simulink model "control_tests"  (R2023b)
settings: Solver=VariableStepAuto  StartTime=0.0  StopTime=30  RelTol=1e-3
values from neighbouring files (symbols this model uses):
  Bp_ = 1.25e-5    (= 1.25e-05)    [stable_pendulum_model.m]
  g_ = 9.81    [stable_pendulum_model.m]
  Jp_ = (1/12)*mp_*(3*rp^2 + Lp^2)    (= 3.3718538025e-05)    [stable_pendulum_model.m]
  Jr_ex_ = 9.5e-5    (= 9.5e-05)    [stable_pendulum_model.m]
  Kc_ = 0.042    [stable_pendulum_model.m]
  Ke_ = 0.042    [stable_pendulum_model.m]
  lp_ = 0.95*Lp/2    (= 0.061275)    [stable_pendulum_model.m]
  Lr_ = 0.09    [stable_pendulum_model.m]
  mp_ = 0.02421    [stable_pendulum_model.m]
  Ra_ = 8.4    [stable_pendulum_model.m]
  theta_0 = 0    [stable_pendulum_model.m]
libraries: cstblocks x3
settings Model: Creator=renzo  LastModifiedBy=renzo

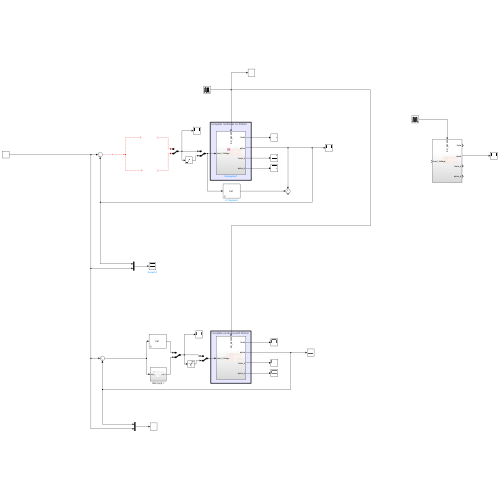
[thumbnail: Simulink's stored preview of the top-level diagram]
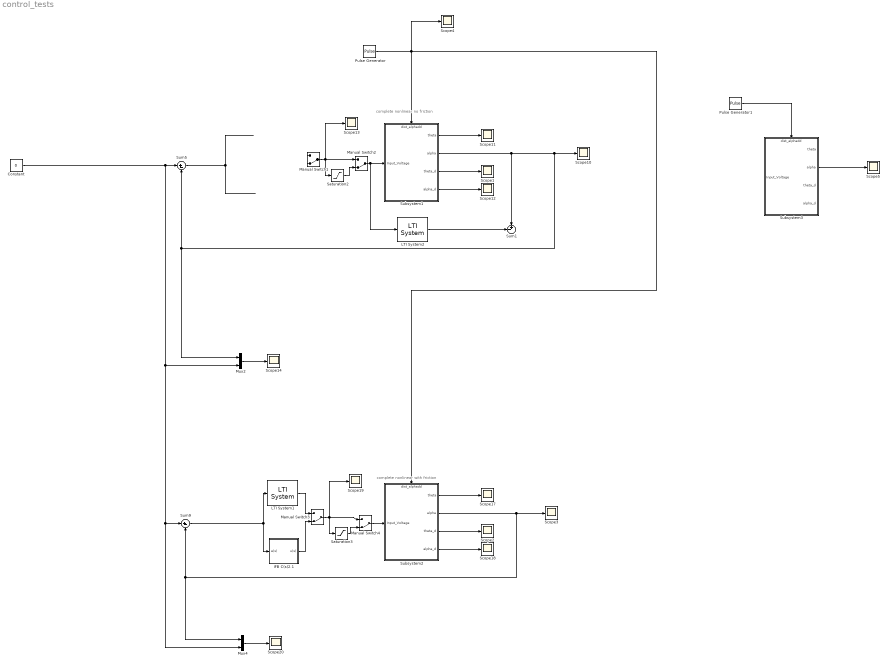
== system control_tests ==
  note: complete nonlinear no friction
  note: complete nonlinear with friction
  Constant : Constant  Value=0
  IFB C(s)2.1 : Subsystem
  LTI System1 : cstblocks/LTI System  sys=Cs1  IC=[]  PadeOrder=0
  LTI System2 : cstblocks/LTI System  sys=Cs1  IC=[]  PadeOrder=0
  Manual Switch{1..4} (4 alike) : ManualSwitch  CurrentSetting=0
  Mux2 : Mux  Inputs=2
  Mux4 : Mux  Inputs=2
  Pulse Generator : DiscretePulseGenerator  PulseType=Time based  Amplitude=20  Period=7  PulseWidth=5  PhaseDelay=3
  Pulse Generator1 : DiscretePulseGenerator  PulseType=Time based  Amplitude=20  Period=7  PulseWidth=5  PhaseDelay=3
  Saturation2 : Saturate  UpperLimit=10  LowerLimit=-10
  Saturation3 : Saturate  UpperLimit=10  LowerLimit=-10
  Scope{1..5,10..14,17..20} (14 alike) : Scope
  Subsystem1 : Subsystem
      settings: PortSchema="{\"entries\":[{\"content\":{\"sides\":[{\"content\":{\"connectorIds\":[\"In1\"]},\"type\":\"ConnectorPlacement.EquallySpacedRectSide\",\"uuid\":\"871ba934-2a41-428b-821f-daa366d85b89\"},{\"content\":{\"connectorIds\":[\"Out1\",\"Out2\",\"Out3\",\"Out4\"],\"side\":\"RIGHT\"},\"type\":\"ConnectorPlacement.EquallySpacedRectSide\",\"uuid\":\"80e9fc77-4911-4b7a-8bf9-66ec4cab57cc\"},{\"content\":{\"connectorIds\":[\"In2\"],\"side\":\"TOP\"},\"type\":\"ConnectorPlacement.EquallySpacedRectSide\",\"uuid\":\"5ed9de82-5230-4695-8afb-09027cc7b06e\"}]},\"type\":\"ConnectorPlacement.EquallySpacedConnector\",\"uuid\":\"352cd2d9-0c64-485c-bb70-89dea2777168\"}],\"packageUris\":[\"http://schema.mathworks.com/mf0/Connector/R2020b\"],\"version\":\"1.0\"}"
  Subsystem2 : Subsystem
      settings: PortSchema="{\"entries\":[{\"content\":{\"sides\":[{\"content\":{\"connectorIds\":[\"In1\"]},\"type\":\"ConnectorPlacement.EquallySpacedRectSide\",\"uuid\":\"871ba934-2a41-428b-821f-daa366d85b89\"},{\"content\":{\"connectorIds\":[\"Out1\",\"Out2\",\"Out3\",\"Out4\"],\"side\":\"RIGHT\"},\"type\":\"ConnectorPlacement.EquallySpacedRectSide\",\"uuid\":\"80e9fc77-4911-4b7a-8bf9-66ec4cab57cc\"},{\"content\":{\"connectorIds\":[\"In2\"],\"side\":\"TOP\"},\"type\":\"ConnectorPlacement.EquallySpacedRectSide\",\"uuid\":\"5ed9de82-5230-4695-8afb-09027cc7b06e\"}]},\"type\":\"ConnectorPlacement.EquallySpacedConnector\",\"uuid\":\"352cd2d9-0c64-485c-bb70-89dea2777168\"}],\"packageUris\":[\"http://schema.mathworks.com/mf0/Connector/R2020b\"],\"version\":\"1.0\"}"
  Subsystem3 : Subsystem
      settings: PortSchema="{\"entries\":[{\"content\":{\"sides\":[{\"content\":{\"connectorIds\":[\"In1\"]},\"type\":\"ConnectorPlacement.EquallySpacedRectSide\",\"uuid\":\"871ba934-2a41-428b-821f-daa366d85b89\"},{\"content\":{\"connectorIds\":[\"Out1\",\"Out2\",\"Out3\",\"Out4\"],\"side\":\"RIGHT\"},\"type\":\"ConnectorPlacement.EquallySpacedRectSide\",\"uuid\":\"80e9fc77-4911-4b7a-8bf9-66ec4cab57cc\"},{\"content\":{\"connectorIds\":[\"In2\"],\"side\":\"TOP\"},\"type\":\"ConnectorPlacement.EquallySpacedRectSide\",\"uuid\":\"5ed9de82-5230-4695-8afb-09027cc7b06e\"}]},\"type\":\"ConnectorPlacement.EquallySpacedConnector\",\"uuid\":\"352cd2d9-0c64-485c-bb70-89dea2777168\"}],\"packageUris\":[\"http://schema.mathworks.com/mf0/Connector/R2020b\"],\"version\":\"1.0\"}"
  Sum1 : Sum  Inputs=-+|
  Sum5 : Sum  Inputs=|+-
  Sum9 : Sum  Inputs=|+-
  wires:
  Mux4/1 -> Scope20/1
  Mux2/1 -> Scope14/1
  Constant/1 -> Mux4/2, Sum9/1, Mux2/2, Sum5/1
  Sum9/1 -> LTI System1/1, IFB C(s)2.1/1(e(s))
  LTI System1/1 -> Manual Switch3/1
  Subsystem1/2(alpha) -> Sum1/2, Sum5/2, Mux2/1, Scope10/1
  Manual Switch4/1 -> Subsystem2/1(Input_Voltage)
  Manual Switch2/1 -> LTI System2/1, Subsystem1/1(Input_Voltage)
  Saturation2/1 -> Manual Switch2/2
  ? -> Manual Switch1/1
  ? -> Manual Switch1/2
  Subsystem2/2(alpha) -> Scope3/1, Sum9/2, Mux4/1
  Subsystem2/1(theta) -> Scope17/1
  IFB C(s)2.1/1(u(s)) -> Manual Switch3/2
  Subsystem2/4(alpha_d) -> Scope18/1
  Manual Switch1/1 -> Saturation2/1, Manual Switch2/1, Scope13/1
  Saturation3/1 -> Manual Switch4/2
  Subsystem1/4(alpha_d) -> Scope12/1
  Manual Switch3/1 -> Saturation3/1, Manual Switch4/1, Scope19/1
  Subsystem1/3(theta_d) -> Scope1/1
  Subsystem1/1(theta) -> Scope11/1
  Sum5/1 -> ?
  Subsystem2/3(theta_d) -> Scope2/1
  Pulse Generator/1 -> Scope4/1, Subsystem2/2(dist_alphadd), Subsystem1/2(dist_alphadd)
  Pulse Generator1/1 -> Subsystem3/2(dist_alphadd)
  Subsystem3/2(alpha) -> Scope5/1
  LTI System2/1 -> Sum1/1

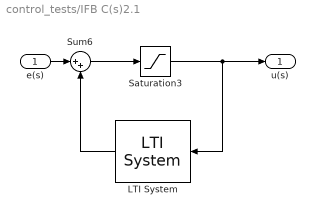
== system control_tests/IFB C(s)2.1 ==
  e(s) : Inport
  LTI System : cstblocks/LTI System  sys=Hs1  IC=[]  PadeOrder=0
  Saturation3 : Saturate  UpperLimit=10  LowerLimit=-10
  Sum6 : Sum  Inputs=|++
  u(s) : Outport
  wires:
  LTI System/1 -> Sum6/2
  Sum6/1 -> Saturation3/1
  Saturation3/1 -> u(s)/1, LTI System/1
  e(s)/1 -> Sum6/1

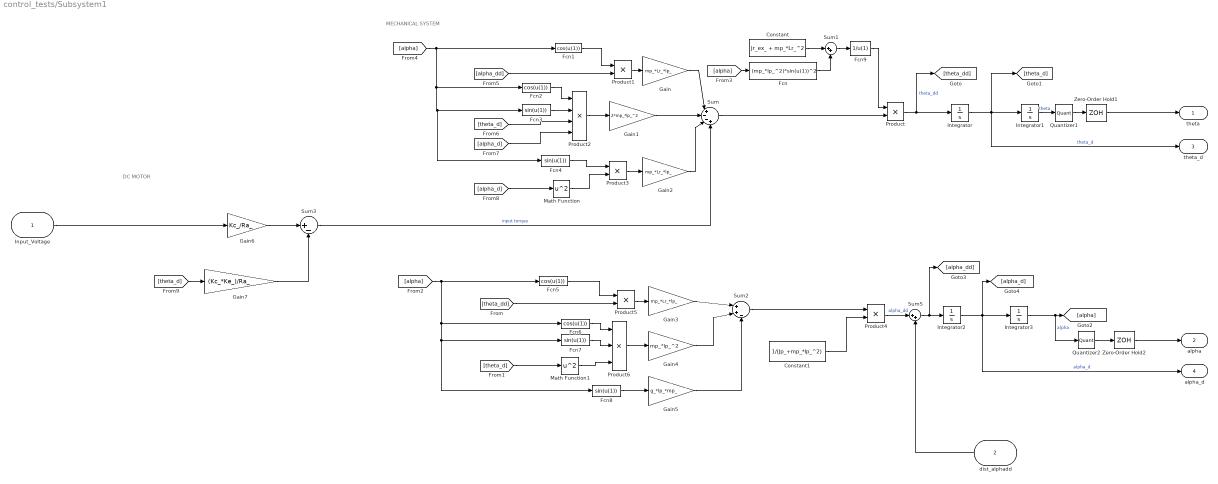
== system control_tests/Subsystem1 ==
  note: DC MOTOR
  note: MECHANICAL SYSTEM
  Input_Voltage : Inport
  dist_alphadd : Inport  Port=2
  Constant : Constant  Value=Jr_ex_ + mp_*Lr_^2
  Constant1 : Constant  Value=1/(Jp_+mp_*lp_^2)
  Fcn : Fcn  Expr=(mp_*lp_^2)*sin(u(1))^2
  Fcn{1..2,5..6} (4 alike) : Fcn  Expr=cos(u(1))
  Fcn{3..4,7..8} (4 alike) : Fcn  Expr=sin(u(1))
  Fcn9 : Fcn  Expr=1/u(1)
  Gain : Gain  Gain=mp_*Lr_*lp_
  Gain1 : Gain  Gain=2*mp_*lp_^2
  Gain2 : Gain  Gain=mp_*Lr_*lp_
  Gain3 : Gain  Gain=mp_*Lr_*lp_
  Gain4 : Gain  Gain=mp_*lp_^2
  Gain5 : Gain  Gain=g_*lp_*mp_
  Gain6 : Gain  Gain=Kc_/Ra_
  Gain7 : Gain  Gain=(Kc_*Ke_)/Ra_
  Integrator : Integrator
  Integrator1 : Integrator  InitialCondition=theta_0
  Integrator2 : Integrator
  Integrator3 : Integrator
  Math Function : Math  Operator=square
  Math Function1 : Math  Operator=square
  Product{,1,3..5} (5 alike) : Product
  Product2 : Product  Inputs=4
  Product6 : Product  Inputs=3
  Quantizer1 : Quantizer  QuantizationInterval=0.0037
  Quantizer2 : Quantizer  QuantizationInterval=0.0037
  Sum : Sum  Inputs=|+--+
  Sum1 : Sum  Inputs=|++
  Sum2 : Sum  Inputs=|++-
  Sum3 : Sum  Inputs=|+-
  Sum5 : Sum  Inputs=|++
  Zero-Order Hold1 : ZeroOrderHold  SampleTime=2e-3
  Zero-Order Hold2 : ZeroOrderHold  SampleTime=2e-3
  theta : Outport
  alpha : Outport  Port=2
  theta_d : Outport  Port=3
  alpha_d : Outport  Port=4
  wires:
  Integrator2/1 -> alpha_d/1, Integrator3/1, [alpha_d]  "alpha_d"
  Fcn6/1 -> Product6/1
  Product4/1 -> Sum5/1  "alpha_dd"
  Fcn4/1 -> Product3/1
  Integrator/1 -> theta_d/1, [theta_d], Integrator1/1  "theta_d"
  Gain1/1 -> Sum/2
  Gain6/1 -> Sum3/1
  Fcn3/1 -> Product2/2
  Fcn1/1 -> Product1/1
  Integrator1/1 -> Quantizer1/1  "theta"
  Fcn8/1 -> Gain5/1
  Fcn7/1 -> Product6/2
  Gain5/1 -> Sum2/3
  Sum1/1 -> Fcn9/1
  Fcn/1 -> Sum1/2
  Product1/1 -> Gain/1
  Fcn9/1 -> Product/1
  Product3/1 -> Gain2/1
  Sum/1 -> Product/2
  [alpha_d] -> Math Function/1
  [theta_dd] -> Product5/2
  [theta_d] -> Gain7/1
  Product5/1 -> Gain3/1
  Fcn5/1 -> Product5/1
  Product6/1 -> Gain4/1
  Sum2/1 -> Product4/1
  Math Function1/1 -> Product6/3
  Math Function/1 -> Product3/2
  Product/1 -> Integrator/1, [theta_dd]  "theta_dd"
  Gain4/1 -> Sum2/2
  Input_Voltage/1 -> Gain6/1
  Constant/1 -> Sum1/1
  [alpha] -> Fcn8/1, Fcn7/1, Fcn6/1, Fcn5/1
  Constant1/1 -> Product4/2
  Product2/1 -> Gain1/1
  [alpha] -> Fcn4/1, Fcn3/1, Fcn2/1, Fcn1/1
  [alpha_d] -> Product2/4
  [alpha_dd] -> Product1/2
  [alpha] -> Fcn/1
  Fcn2/1 -> Product2/1
  Sum3/1 -> Sum/4  "input torque"
  Gain2/1 -> Sum/3
  Gain/1 -> Sum/1
  Gain3/1 -> Sum2/1
  [theta_d] -> Math Function1/1
  Gain7/1 -> Sum3/2
  [theta_d] -> Product2/3
  Quantizer1/1 -> Zero-Order Hold1/1
  Zero-Order Hold1/1 -> theta/1
  Quantizer2/1 -> Zero-Order Hold2/1
  Zero-Order Hold2/1 -> alpha/1
  Integrator3/1 -> Quantizer2/1, [alpha]  "alpha"
  Sum5/1 -> [alpha_dd], Integrator2/1
  dist_alphadd/1 -> Sum5/2

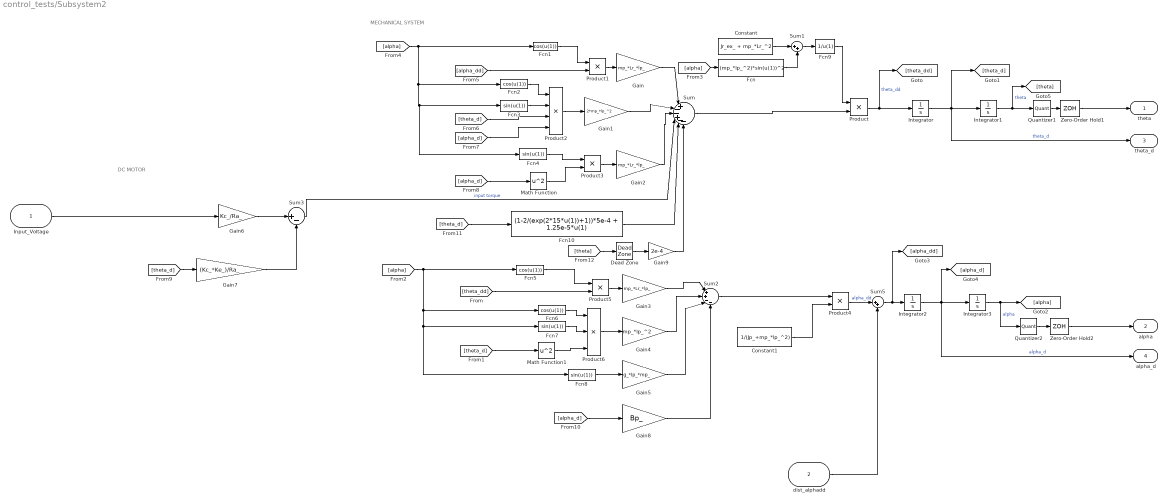
== system control_tests/Subsystem2 ==
  note: MECHANICAL SYSTEM
  note: DC MOTOR
  Input_Voltage : Inport
  dist_alphadd : Inport  Port=2
  Constant : Constant  Value=Jr_ex_ + mp_*Lr_^2
  Constant1 : Constant  Value=1/(Jp_+mp_*lp_^2)
  Dead Zone : DeadZone  LowerValue=0  UpperValue=0  ZeroCross=off
  Fcn : Fcn  Expr=(mp_*lp_^2)*sin(u(1))^2
  Fcn{1..2,5..6} (4 alike) : Fcn  Expr=cos(u(1))
  Fcn10 : Fcn  Expr=(1-2/(exp(2*15*u(1))+1))*5e-4 + 1.25e-5*u(1)
  Fcn{3..4,7..8} (4 alike) : Fcn  Expr=sin(u(1))
  Fcn9 : Fcn  Expr=1/u(1)
  Gain : Gain  Gain=mp_*Lr_*lp_
  Gain1 : Gain  Gain=2*mp_*lp_^2
  Gain2 : Gain  Gain=mp_*Lr_*lp_
  Gain3 : Gain  Gain=mp_*Lr_*lp_
  Gain4 : Gain  Gain=mp_*lp_^2
  Gain5 : Gain  Gain=g_*lp_*mp_
  Gain6 : Gain  Gain=Kc_/Ra_
  Gain7 : Gain  Gain=(Kc_*Ke_)/Ra_
  Gain8 : Gain  Gain=Bp_
  Gain9 : Gain  Gain=2e-4
  Integrator{,1..3} (4 alike) : Integrator
  Math Function : Math  Operator=square
  Math Function1 : Math  Operator=square
  Product{,1,3..5} (5 alike) : Product
  Product2 : Product  Inputs=4
  Product6 : Product  Inputs=3
  Quantizer1 : Quantizer  QuantizationInterval=0.0037
  Quantizer2 : Quantizer  QuantizationInterval=0.0037
  Sum : Sum  Inputs=|+--+--
  Sum1 : Sum  Inputs=|++
  Sum2 : Sum  Inputs=|++--
  Sum3 : Sum  Inputs=|+-
  Sum5 : Sum  Inputs=|++
  Zero-Order Hold1 : ZeroOrderHold  SampleTime=2e-3
  Zero-Order Hold2 : ZeroOrderHold  SampleTime=2e-3
  theta : Outport
  alpha : Outport  Port=2
  theta_d : Outport  Port=3
  alpha_d : Outport  Port=4
  wires:
  [theta_d] -> Product2/3
  Gain7/1 -> Sum3/2
  [theta_d] -> Math Function1/1
  Gain3/1 -> Sum2/1
  Gain/1 -> Sum/1
  Gain2/1 -> Sum/3
  Sum3/1 -> Sum/4  "input torque"
  Fcn2/1 -> Product2/1
  [alpha] -> Fcn/1
  [alpha_dd] -> Product1/2
  [alpha_d] -> Product2/4
  [alpha] -> Fcn1/1, Fcn2/1, Fcn3/1, Fcn4/1
  Product2/1 -> Gain1/1
  Constant1/1 -> Product4/2
  [alpha] -> Fcn5/1, Fcn6/1, Fcn7/1, Fcn8/1
  Constant/1 -> Sum1/1
  Input_Voltage/1 -> Gain6/1
  Gain4/1 -> Sum2/2
  Product/1 -> [theta_dd], Integrator/1  "theta_dd"
  Math Function/1 -> Product3/2
  Math Function1/1 -> Product6/3
  Sum2/1 -> Product4/1
  Product6/1 -> Gain4/1
  Fcn5/1 -> Product5/1
  Integrator3/1 -> [alpha], Quantizer2/1  "alpha"
  Product5/1 -> Gain3/1
  [theta_d] -> Gain7/1
  [theta_dd] -> Product5/2
  [alpha_d] -> Math Function/1
  Sum/1 -> Product/2
  Product3/1 -> Gain2/1
  Fcn9/1 -> Product/1
  Product1/1 -> Gain/1
  Fcn/1 -> Sum1/2
  Sum1/1 -> Fcn9/1
  Gain5/1 -> Sum2/3
  Fcn7/1 -> Product6/2
  Fcn8/1 -> Gain5/1
  Integrator1/1 -> Quantizer1/1, [theta]  "theta"
  Fcn1/1 -> Product1/1
  Fcn3/1 -> Product2/2
  Gain6/1 -> Sum3/1
  Gain1/1 -> Sum/2
  Integrator/1 -> Integrator1/1, [theta_d], theta_d/1  "theta_d"
  Fcn4/1 -> Product3/1
  Product4/1 -> Sum5/1  "alpha_dd"
  Fcn6/1 -> Product6/1
  Integrator2/1 -> [alpha_d], Integrator3/1, alpha_d/1  "alpha_d"
  [alpha_d] -> Gain8/1
  Gain8/1 -> Sum2/4
  [theta_d] -> Fcn10/1
  Dead Zone/1 -> Gain9/1
  Gain9/1 -> Sum/6
  [theta] -> Dead Zone/1
  Fcn10/1 -> Sum/5
  Quantizer1/1 -> Zero-Order Hold1/1
  Zero-Order Hold1/1 -> theta/1
  Quantizer2/1 -> Zero-Order Hold2/1
  Zero-Order Hold2/1 -> alpha/1
  Sum5/1 -> [alpha_dd], Integrator2/1
  dist_alphadd/1 -> Sum5/2

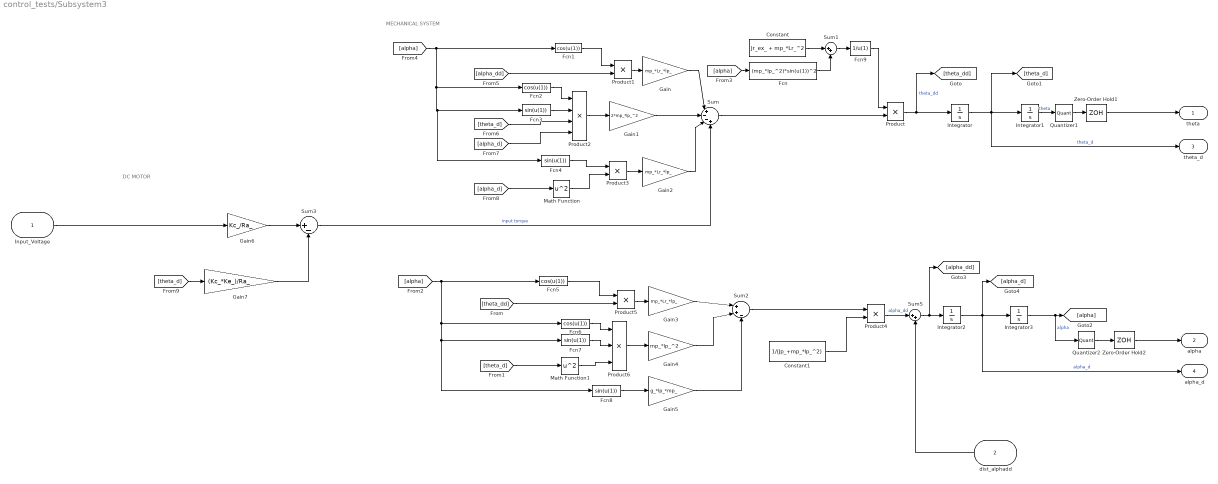
== system control_tests/Subsystem3 ==
  note: MECHANICAL SYSTEM
  note: DC MOTOR
  Input_Voltage : Inport
  dist_alphadd : Inport  Port=2
  Constant : Constant  Value=Jr_ex_ + mp_*Lr_^2
  Constant1 : Constant  Value=1/(Jp_+mp_*lp_^2)
  Fcn : Fcn  Expr=(mp_*lp_^2)*sin(u(1))^2
  Fcn{1..2,5..6} (4 alike) : Fcn  Expr=cos(u(1))
  Fcn{3..4,7..8} (4 alike) : Fcn  Expr=sin(u(1))
  Fcn9 : Fcn  Expr=1/u(1)
  Gain : Gain  Gain=mp_*Lr_*lp_
  Gain1 : Gain  Gain=2*mp_*lp_^2
  Gain2 : Gain  Gain=mp_*Lr_*lp_
  Gain3 : Gain  Gain=mp_*Lr_*lp_
  Gain4 : Gain  Gain=mp_*lp_^2
  Gain5 : Gain  Gain=g_*lp_*mp_
  Gain6 : Gain  Gain=Kc_/Ra_
  Gain7 : Gain  Gain=(Kc_*Ke_)/Ra_
  Integrator : Integrator
  Integrator1 : Integrator  InitialCondition=theta_0
  Integrator2 : Integrator
  Integrator3 : Integrator
  Math Function : Math  Operator=square
  Math Function1 : Math  Operator=square
  Product{,1,3..5} (5 alike) : Product
  Product2 : Product  Inputs=4
  Product6 : Product  Inputs=3
  Quantizer1 : Quantizer  QuantizationInterval=0.0037
  Quantizer2 : Quantizer  QuantizationInterval=0.0037
  Sum : Sum  Inputs=|+--+
  Sum1 : Sum  Inputs=|++
  Sum2 : Sum  Inputs=|++-
  Sum3 : Sum  Inputs=|+-
  Sum5 : Sum  Inputs=|++
  Zero-Order Hold1 : ZeroOrderHold  SampleTime=2e-3
  Zero-Order Hold2 : ZeroOrderHold  SampleTime=2e-3
  theta : Outport
  alpha : Outport  Port=2
  theta_d : Outport  Port=3
  alpha_d : Outport  Port=4
  wires:
  dist_alphadd/1 -> Sum5/2
  Sum5/1 -> Integrator2/1, [alpha_dd]
  Integrator3/1 -> [alpha], Quantizer2/1  "alpha"
  Zero-Order Hold2/1 -> alpha/1
  Quantizer2/1 -> Zero-Order Hold2/1
  Zero-Order Hold1/1 -> theta/1
  Quantizer1/1 -> Zero-Order Hold1/1
  [theta_d] -> Product2/3
  Gain7/1 -> Sum3/2
  [theta_d] -> Math Function1/1
  Gain3/1 -> Sum2/1
  Gain/1 -> Sum/1
  Gain2/1 -> Sum/3
  Sum3/1 -> Sum/4  "input torque"
  Fcn2/1 -> Product2/1
  [alpha] -> Fcn/1
  [alpha_dd] -> Product1/2
  [alpha_d] -> Product2/4
  [alpha] -> Fcn1/1, Fcn2/1, Fcn3/1, Fcn4/1
  Product2/1 -> Gain1/1
  Constant1/1 -> Product4/2
  [alpha] -> Fcn5/1, Fcn6/1, Fcn7/1, Fcn8/1
  Constant/1 -> Sum1/1
  Input_Voltage/1 -> Gain6/1
  Gain4/1 -> Sum2/2
  Product/1 -> [theta_dd], Integrator/1  "theta_dd"
  Math Function/1 -> Product3/2
  Math Function1/1 -> Product6/3
  Sum2/1 -> Product4/1
  Product6/1 -> Gain4/1
  Fcn5/1 -> Product5/1
  Product5/1 -> Gain3/1
  [theta_d] -> Gain7/1
  [theta_dd] -> Product5/2
  [alpha_d] -> Math Function/1
  Sum/1 -> Product/2
  Product3/1 -> Gain2/1
  Fcn9/1 -> Product/1
  Product1/1 -> Gain/1
  Fcn/1 -> Sum1/2
  Sum1/1 -> Fcn9/1
  Gain5/1 -> Sum2/3
  Fcn7/1 -> Product6/2
  Fcn8/1 -> Gain5/1
  Integrator1/1 -> Quantizer1/1  "theta"
  Fcn1/1 -> Product1/1
  Fcn3/1 -> Product2/2
  Gain6/1 -> Sum3/1
  Gain1/1 -> Sum/2
  Integrator/1 -> Integrator1/1, [theta_d], theta_d/1  "theta_d"
  Fcn4/1 -> Product3/1
  Product4/1 -> Sum5/1  "alpha_dd"
  Fcn6/1 -> Product6/1
  Integrator2/1 -> [alpha_d], Integrator3/1, alpha_d/1  "alpha_d"
